simulink model "DC_Motor_Openloop_Speed_Monitoring"  (R2024b)
settings: Solver=FixedStepDiscrete  StartTime=0.0  StopTime=inf  FixedStep=0.01  RelTol=1e-3
libraries: arduinolib x3, arduinosensorlib x1
settings Model: Creator=Nabil  LastModifiedBy=Nabil
settings SolverCC: AutoInsertRateTranBlk=on
settings OptimizationCC: EnhancedBackFolding=on  PassReuseOutputArgsAs=Individual arguments  ZeroExternalMemoryAtStartup=off  ZeroInternalMemoryAtStartup=off  MaxStackSize=64  OptimizeBlockOrder=speed  DifferentSizesBufferReuse=on  OptimizationCustomize=off  EfficientTunableParamExpr=on
settings DebuggingCC: ParameterTunabilityLossMsg=error
settings HardwareCC: ProdBitPerInt=16  ProdBitPerPointer=16  ProdBitPerSizeT=16  ProdBitPerPtrDiffT=16  ProdLargestAtomicFloat=None  ProdWordSize=8  ProdHWDeviceType=Atmel->AVR
settings SFSimCC: MATLABDynamicMemAlloc=off
settings RTWCC: Description=Embedded Coder  SystemTargetFile=ert.tlc  HardwareBoard=Arduino Uno  TemplateMakefile=ert_default_tmf  Toolchain=Arduino AVR
settings CodeAppCC: ForceParamTrailComments=on  IgnoreCustomStorageClasses=off  OperatorAnnotations=on  SimulinkDataObjDesc=on  SFDataObjDesc=on  InsertBlockDesc=on
settings ERTTargetCC: SupportContinuousTime=on  SupportVariableSizeSignals=on  ExtModeTransport=3  ExtModeStaticAlloc=on  ExtModeAutomaticAllocSize=off  ExtModeStaticAllocSize=250  ExtModeMexFile=ext_xcp  ExtModeIntrfLevel=Level2 - Open  InlinedParameterPlacement=Hierarchical

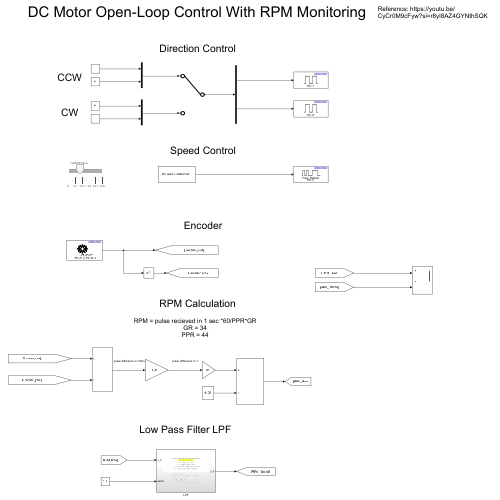
[thumbnail: Simulink's stored preview of the top-level diagram]
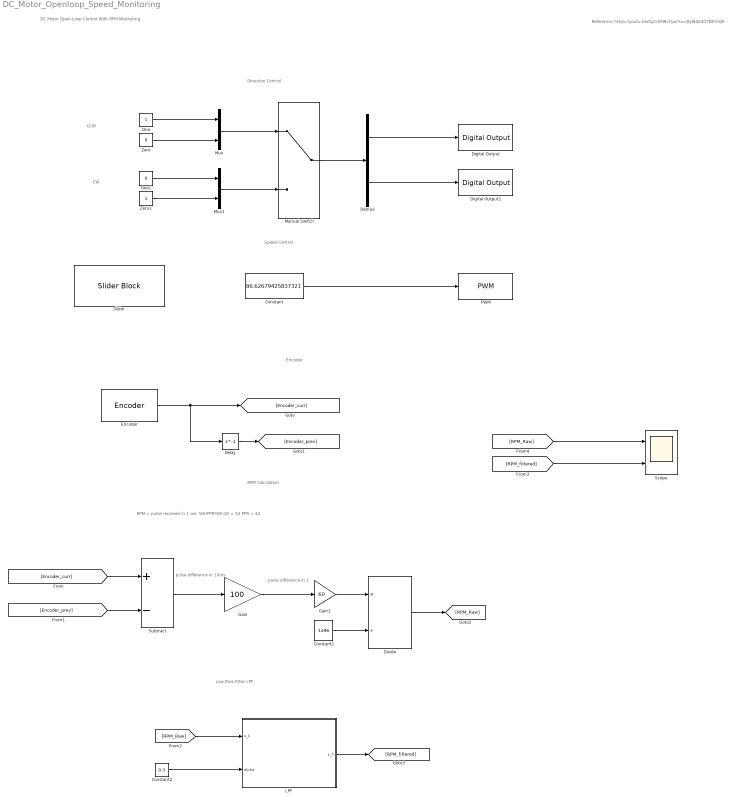
== system DC_Motor_Openloop_Speed_Monitoring ==
  note: Reference: https://youtu.be/CyCr0M9cFyw?si=r8yl8AZ4GYNthSQK
  note: pulse difference in 10ms
  note: DC Motor Open-Loop Control With RPM Monitoring
  note: Direction Control
  note: CCW
  note: Speed Control
  note: CW
  note: Encoder
  note: RPM Calculation
  note: RPM = pulse recieved in 1 sec *60/PPR*GR
      | GR = 34
      | PPR = 44
  note: pulse difference in 1
  note: Low Pass Filter LPF
  Constant : Constant  Value=86.62679425837321  OutMin=0  OutMax=255  OutDataTypeStr=uint8
  Constant1 : Constant  Value=1496
  Constant2 : Constant  Value=0.3
  Delay : Delay  DelayLength=1  InputProcessing=Columns as channels (frame based)
  Demux : Demux  Outputs=2
  Digital Output : arduinolib/Digital Output  pinNumber=7  Direction=output  blockPlatform=arduino
      settings: SourceProductName=Common
  Digital Output1 : arduinolib/Digital Output  pinNumber=6  Direction=output  blockPlatform=arduino
      settings: SourceProductName=Common
  Divide : Product  Inputs=*/
  Encoder : arduinosensorlib/Encoder  InputA=2  InputB=3  Mode=No reset  SampleTime=-1
      settings: SourceProductName=Sensors
  Gain : Gain  Gain=100
  Gain1 : Gain  Gain=60
  LPF : Subsystem
  Manual Switch : ManualSwitch
  Mux : Mux  Inputs=2
  Mux1 : Mux  Inputs=2
  One : Constant  OutDataTypeStr=uint8
  One1 : Constant  Value=0  OutDataTypeStr=Inherit: Inherit via back propagation
  PWM : arduinolib/PWM  pinNumber=5  frequencyType=Default  desiredFrequency=490.2  achievableFrequency=490.2
      settings: SourceProductName=Common
  Scope : Scope  NumInputPorts=2
  Slider : SliderBlock  ScaleMax=255
  Subtract : Sum  Inputs=+-
  Zero : Constant  Value=0  OutDataTypeStr=uint8
  Zero1 : Constant  OutDataTypeStr=Inherit: Inherit via back propagation
  wires:
  One1/1 -> Mux1/1
  Zero1/1 -> Mux1/2
  Constant/1 -> PWM/1
  Encoder/1 -> [Encoder_curr], Delay/1
  Delay/1 -> [Encoder_prev]
  [Encoder_prev] -> Subtract/2
  [Encoder_curr] -> Subtract/1
  Subtract/1 -> Gain/1
  Gain/1 -> Gain1/1
  Gain1/1 -> Divide/1
  Constant1/1 -> Divide/2
  Divide/1 -> [RPM_Raw]
  [RPM_Raw] -> LPF/1(x_k)
  Constant2/1 -> LPF/2(alpha)
  LPF/1(y_k) -> [RPM_filtered]
  Zero/1 -> Mux/2
  One/1 -> Mux/1
  Mux/1 -> Manual Switch/1
  Mux1/1 -> Manual Switch/2
  Manual Switch/1 -> Demux/1
  Demux/1 -> Digital Output/1
  Demux/2 -> Digital Output1/1
  [RPM_Raw] -> Scope/1
  [RPM_filtered] -> Scope/2

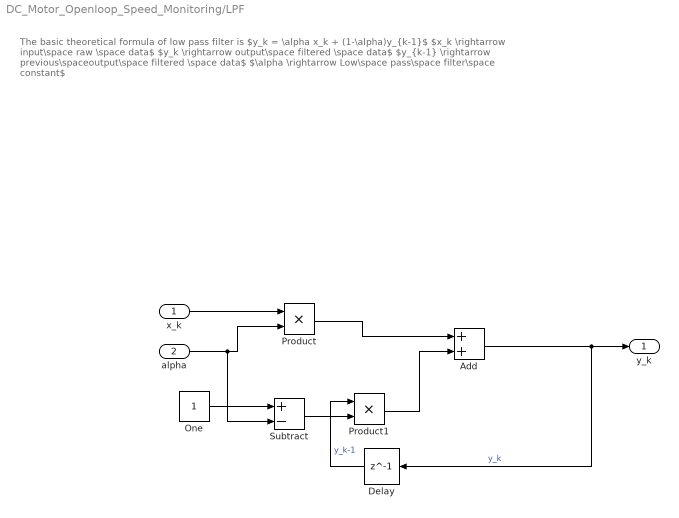
== system DC_Motor_Openloop_Speed_Monitoring/LPF ==
  note: The basic theoretical formula of low pass filter is
      | $y_k = \alpha x_k + (1-\alpha)y_{k-1}$
      | $x_k \rightarrow input\space raw \space data$
      | $y_k \rightarrow output\space filtered \space data$
      | $y_{k-1} \rightarrow previous\spaceoutput\space filtered \space data$
      | $\alpha \rightarrow Low\space pass\space filter\space constant$
  x_k : Inport
  alpha : Inport  Port=2
  Add : Sum
  Delay : Delay  DelayLength=1  InputProcessing=Columns as channels (frame based)
  One : Constant  OutDataTypeStr=Inherit: Inherit via back propagation
  Product : Product
  Product1 : Product
  Subtract : Sum  Inputs=+-
  y_k : Outport
  wires:
  x_k/1 -> Product/1
  alpha/1 -> Subtract/2, Product/2
  Product/1 -> Add/1
  Add/1 -> Delay/1, y_k/1  "y_k"
  One/1 -> Subtract/1
  Subtract/1 -> Product1/2
  Delay/1 -> Product1/1  "y_k-1"
  Product1/1 -> Add/2
